simulink model "resetteble_test1"  (R2022b)
settings: Solver=VariableStepAuto  StartTime=0.0  StopTime=10.0  RelTol=1e-3
undefined symbols (not defined in the file or in its folder): DiscIntNeverNeededParam
libraries: simulink x1
settings Model: Creator=hp_desktop  LastModifiedBy=hp_desktop

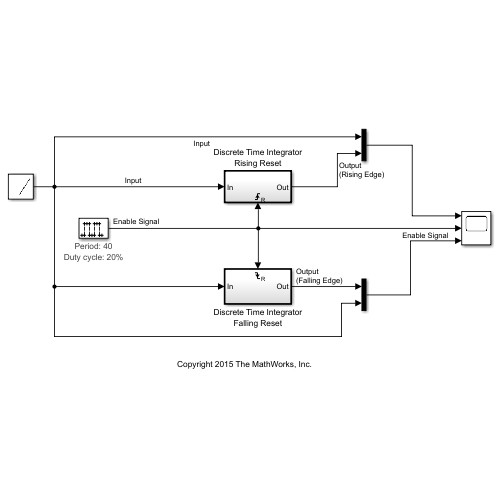
[thumbnail: Simulink's stored preview of the top-level diagram]
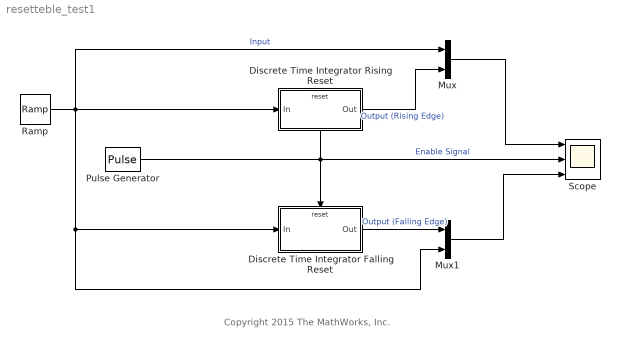
== system resetteble_test1 ==
  note: Copyright 2015 The MathWorks, Inc.
  Discrete Time Integrator Falling Reset : Subsystem  TreatAsAtomicUnit=on
  Discrete Time Integrator Rising Reset : Subsystem  TreatAsAtomicUnit=on
  Mux : Mux  Inputs=2
  Mux1 : Mux  Inputs=2
  Pulse Generator : DiscretePulseGenerator  Period=40  PulseWidth=20  SampleTime=.1
      settings: AttributesFormatString=Period: %<period>\nDuty cycle: %<pulsewidth>%
  Ramp : simulink/Sources/Ramp  slope=0.5  start=0  InitialOutput=1
  Scope : Scope  NumInputPorts=3
      settings: StartFcn=open_system(gcbh)
  wires:
  Pulse Generator/1 -> Scope/2, Discrete Time Integrator Falling Reset/Reset, Discrete Time Integrator Rising Reset/Reset  "Enable Signal"
  Mux1/1 -> Scope/3
  Discrete Time Integrator Falling Reset/1(Out) -> Mux1/1  "Output (Falling Edge)"
  Mux/1 -> Scope/1
  Ramp/1 -> Mux/1, Discrete Time Integrator Rising Reset/1(In), Mux1/2, Discrete Time Integrator Falling Reset/1(In)  "Input"
  Discrete Time Integrator Rising Reset/1(Out) -> Mux/2  "Output (Rising Edge)"

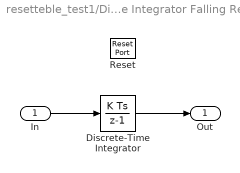
== system resetteble_test1/Discrete Time Integrator Falling Reset ==
  In : Inport  SampleTime=.1
  Reset : ResetPort  DisableCoverage=on  ResetTriggerType=falling
  Discrete-Time Integrator : DiscreteIntegrator  SampleTime=.1  ICPrevOutput=DiscIntNeverNeededParam  ICPrevScaledInput=DiscIntNeverNeededParam
  Out : Outport  VectorParamsAs1DForOutWhenUnconnected=off
  wires:
  Discrete-Time Integrator/1 -> Out/1
  In/1 -> Discrete-Time Integrator/1

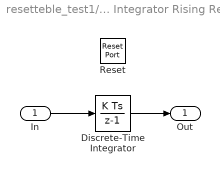
== system resetteble_test1/Discrete Time Integrator Rising Reset ==
  In : Inport  SampleTime=0.1
  Reset : ResetPort  DisableCoverage=on
  Discrete-Time Integrator : DiscreteIntegrator  SampleTime=-1  ICPrevOutput=DiscIntNeverNeededParam  ICPrevScaledInput=DiscIntNeverNeededParam
  Out : Outport  OutputWhenDisabled=reset  InitialOutput=0  VectorParamsAs1DForOutWhenUnconnected=off
  wires:
  In/1 -> Discrete-Time Integrator/1
  Discrete-Time Integrator/1 -> Out/1
